simulink library "Yaw_Motor_Lib"  (Simulink 7.9)
settings: Solver=ode45  StartTime=0.0  StopTime=10.0  RelTol=1e-3
undefined symbols (not defined in the file): deg, gcbh, mech_rtmsupport, mech_support, s, WT_Params
libraries: fl_lib x7, mblibv1 x6, nesl_utility x5, elec_lib x1, Yaw_Gearbox_Lib x1
Description:
  | Copyright 2011 MathWorks, Inc.
settings Model: Creator=smiller  LastModifiedBy=smiller

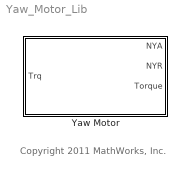
== system Yaw_Motor_Lib ==
  note: Copyright 2011 MathWorks, Inc.
  Yaw Motor : Subsystem
      mask Display: image(imread('Yaw_Servomotor_Horizontal_IMAGE.jpg'));

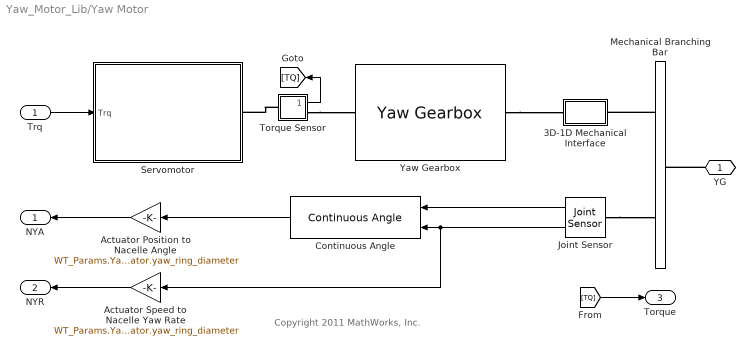
== system Yaw_Motor_Lib/Yaw Motor ==
  note: Copyright 2011 MathWorks, Inc.
  Trq : Inport
  3D-1D Mechanical Interface : Subsystem
  Actuator Position to Nacelle Angle : Gain  Gain=WT_Params.Yaw_Actuator.yaw_gear_diameter/WT_Params.Yaw_Actuator.yaw_ring_diameter
  Actuator Speed to Nacelle Yaw Rate : Gain  Gain=WT_Params.Yaw_Actuator.yaw_gear_diameter/WT_Params.Yaw_Actuator.yaw_ring_diameter
  Continuous Angle : mblibv1/Utilities/Continuous Angle  rad=deg  rads=deg/s
  Joint Sensor : mblibv1/Sensors &  Actuators/Joint Sensor  UpdateFromCAD=off  PhysicalDomain=Mechanical  PortType=blob  Muxed=off  Pose=off  Angle=on  AngleUnits=deg  ArcVelocity=on  ArcVelocityUnits=deg/s  ArcAcceleration=off  ArcAccelerationUnits=deg/s^2  CoordPosition=on  CoordPositionUnits=m  Velocity=off  VelocityUnits=m/s  Acceleration=off  AccelerationUnits=m/s^2  Quaternion=on  QuaternionDT=off  QuaternionDDT=off  QuaternionUnits=off  OutputVector=[1]  ActiveIO=off  Width=2  DialogClass=MechanicalSensorBlock  Primitive=R1  Force=off  ForceUnits=N  Torque=off  TorqueUnits=N*m  ReferenceFrame=Absolute (World)  ReactionSensedSide=Base  ReactionReferenceFrame=Local (Body CS)  ReactionForce=off  ReactionForceUnits=N  ReactionMoment=off  ReactionMomentUnits=N*m
  Mechanical Branching Bar : mblibv1/Utilities/Mechanical Branching Bar  LConnTagsString=_newl0  RConnTagsString=SA0|SA1  UpdateFromCAD=off  DialogClass=MechanicalBranchingBarBlock  NumSAPorts=2
  Servomotor : Subsystem
      mask Display: image(imread('Yaw_Servomotor_IMAGE.jpg'));
  Torque Sensor : Subsystem
      mask Display: disp('S')
  Yaw Gearbox : Yaw_Gearbox_Lib/Yaw Gearbox  SystemSampleTime=-1
  YG : PMIOPort  Port=1  Side=Right
  NYA : Outport
  NYR : Outport  Port=2
  Torque : Outport  Port=3
  wires:
  Trq/1 -> Servomotor/1(Trq)
  Joint Sensor/2 -> Actuator Speed to Nacelle Yaw Rate/1, Continuous Angle/2
  Joint Sensor/1 -> Continuous Angle/1
  Continuous Angle/1 -> Actuator Position to Nacelle Angle/1
  Actuator Position to Nacelle Angle/1 -> NYA/1
  Actuator Speed to Nacelle Yaw Rate/1 -> NYR/1
  Torque Sensor/1(Trq) -> [TQ]
  [TQ] -> Torque/1
  connections:
  Mechanical Branching Bar/RConn1 -- 3D-1D Mechanical Interface/RConn1
  Joint Sensor/LConn1 -- Mechanical Branching Bar/RConn2
  YG/RConn1 -- Mechanical Branching Bar/LConn1
  Torque Sensor/LConn1 -- Servomotor/RConn1
  Torque Sensor/RConn1 -- Yaw Gearbox/LConn1
  Yaw Gearbox/RConn1 -- 3D-1D Mechanical Interface/LConn1

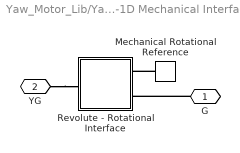
== system Yaw_Motor_Lib/Yaw Motor/3D-1D Mechanical Interface ==
  Mechanical Rotational Reference : fl_lib/Mechanical/Rotational Elements/Mechanical Rotational Reference  t_Log=off  LocalVarNames=|t  LocalVarDescs=|t  LocalVarLogging=0
  Revolute - Rotational Interface : Subsystem  DialogController=MECH.DynMechDlgSource  LoadFcn=mech_rtmsupport('LoadFcn',gcbh);mech_support('LoadFcn',gcbh);  StartFcn=mech_support('StartFcn',gcbh);  StopFcn=mech_support('StopFcn',gcbh);  mask(Revolute - Rotational Interface){UpdateFromCAD=off, PMImportedID=, ClassName=RevoluteRotationalInterface, DialogClass=RevoluteRotationalInterface, Primitive=R1}
      mask prompts: UpdateFromCAD "UPDATE_FROM_CAD"; PMImportedID "PMIMPORTED_ID"; Primitive "Connected to primitive :"
      mask help:
      | Connects a revolute primitive in the Joint attached at port R to any two mechanical rotational nodes in a Simscape network. Exchanges rotational kinetic energy between a machine and a network without loss. The base (B) and follower (F) ports correspond to the same ports on the Joint. Connect to Joint block to see Connected to primitive list.
      |
      | To ensure model validity, do not place inertia elements in interfaced Simscape circuit.
      mask init:
      | mech_preinitmask ();
      | mech_support('MaskInit',gcbh)
      settings: CopyFcn=mech_rtmsupport('CopyFcn',gcbh);mech_support('CopyFcn',gcbh);  DeleteFcn=mech_rtmsupport('DeleteFcn',gcbh);mech_support('DeleteFcn',gcbh);  UndoDeleteFcn=mech_support('UndoDeleteFcn',gcbh);  ModelCloseFcn=mech_rtmsupport('ModelCloseFcn',gcbh);mech_support('ModelCloseFcn',gcbh);  PreSaveFcn=mech_rtmsupport('PreSaveFcn',gcbh);  PostSaveFcn=mech_rtmsupport('PostSaveFcn',gcbh);  NameChangeFcn=mech_support('NameChangeFcn',gcbh);  PreCopyFcn=mech_rtmsupport('PreCopyFcn',gcbh);  CloseFcn=mech_support('CloseFcn',gcbh);  PreDeleteFcn=mech_rtmsupport('PreDeleteFcn',gcbh);
      mask Help: web(mech_help('revoluterotationalinterface'))
      mask Display: image(mech_getIcon('revolute_interface.bmp', 'Mechanical'),'center','on');color('magenta');port_label('lconn',1,'B');port_label('lconn',2,'F');color('black');port_label('rconn',1,'R');
  G : PMIOPort  Port=1  Side=Left
  YG : PMIOPort  Port=2  Side=Right
  connections:
  G/RConn1 -- Revolute - Rotational Interface/LConn2
  Mechanical Rotational Reference/LConn1 -- Revolute - Rotational Interface/LConn1
  YG/RConn1 -- Revolute - Rotational Interface/RConn1

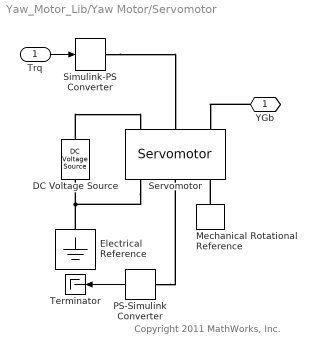
== system Yaw_Motor_Lib/Yaw Motor/Servomotor ==
  note: Copyright 2011 MathWorks, Inc.
  Trq : Inport
  DC Voltage Source : fl_lib/Electrical/Electrical Sources/DC Voltage Source  v0=WT_Params.Yaw_Actuator.Motor.voltage V  i_Log=off  v_Log=off  LocalVarNames=|current|voltage|power  LocalVarDescs=|Current (A)|Voltage (V)|Power (W)  LocalVarLogging=[0 0 0]
  Electrical Reference : fl_lib/Electrical/Electrical Elements/Electrical Reference  i_Log=off  LocalVarNames=|i  LocalVarDescs=|i  LocalVarLogging=[]
  Mechanical Rotational Reference : fl_lib/Mechanical/Rotational Elements/Mechanical Rotational Reference  t_Log=off  LocalVarNames=|t  LocalVarDescs=|t  LocalVarLogging=[]
  PS-Simulink Converter : nesl_utility/PS-Simulink Converter  PhysicalDomain=network_engine_domain  LeftPortType=input  RightPortType=output  SubClassName=ps_output  Unit=deg/s  AffineConversion=off
  Servomotor : elec_lib/Actuators & Drivers/Rotational Actuators/Servomotor  w_t=WT_Params.Yaw_Actuator.Motor.max_speed_vector  T_t=WT_Params.Yaw_Actuator.Motor.max_torque_vector  Tc=WT_Params.Yaw_Actuator.Motor.control_time_constant s  eff=100  w_eff=3.75e+03 rpm  T_eff=0.08 N*m  Pbase=0 W  Res=WT_Params.Yaw_Actuator.Motor.resistance Ohm  J=0 kg*m^2  lam=WT_Params.Yaw_Actuator.Motor.damping N*m/(rad/s)  speed0=0 rpm  LocalVarLogging=[]  alpha=0.00393 1/K  Tmeas=25 C  thermal_mass=100 J/K  initial_temperature=25 C
  Simulink-PS Converter : nesl_utility/Simulink-PS Converter  PhysicalDomain=network_engine_domain  LeftPortType=input  RightPortType=output  SubClassName=ps_input  Unit=1  AffineConversion=off  InputFilterTimeConstant=.001  UdotUserProvided=0  SimscapeFilterOrder=1  InputFiltering=off
  Terminator : Terminator
  YGb : PMIOPort  Port=1  Side=Right
  wires:
  PS-Simulink Converter/1 -> Terminator/1
  Trq/1 -> Simulink-PS Converter/1
  connections:
  DC Voltage Source/LConn1 -- Servomotor/LConn1
  Servomotor/RConn1 -- DC Voltage Source/RConn1 -- Electrical Reference/LConn1
  Mechanical Rotational Reference/LConn1 -- Servomotor/RConn3
  PS-Simulink Converter/LConn1 -- Servomotor/RConn2
  Simulink-PS Converter/RConn1 -- Servomotor/LConn2
  YGb/RConn1 -- Servomotor/LConn3

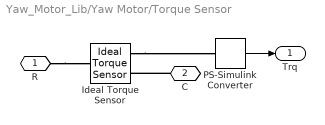
== system Yaw_Motor_Lib/Yaw Motor/Torque Sensor ==
  Ideal Torque Sensor : fl_lib/Mechanical/Mechanical Sensors/Ideal Torque Sensor  w_Log=off  t_Log=off  LocalVarNames=|w|t  LocalVarDescs=|w|t  LocalVarLogging=[0 0]
  PS-Simulink Converter : nesl_utility/PS-Simulink Converter  SystemSampleTime=-1  PhysicalDomain=network_engine_domain  LeftPortType=input  RightPortType=output  SubClassName=ps_output  Unit=1  AffineConversion=off
  R : PMIOPort  Port=1  Side=Left
  C : PMIOPort  Port=2  Side=Right
  Trq : Outport
  wires:
  PS-Simulink Converter/1 -> Trq/1
  connections:
  R/RConn1 -- Ideal Torque Sensor/LConn1
  C/RConn1 -- Ideal Torque Sensor/RConn1
  Ideal Torque Sensor/RConn2 -- PS-Simulink Converter/LConn1

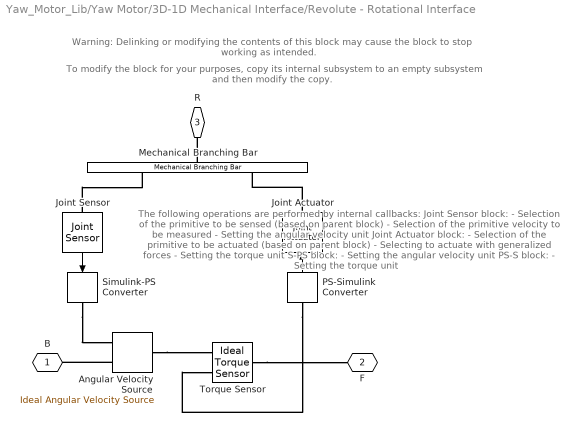
== system Yaw_Motor_Lib/Yaw Motor/3D-1D Mechanical Interface/Revolute - Rotational Interface ==
  note: Warning: Delinking or modifying the contents of
      | this block may cause the block to stop working as intended.
  note: To modify the block for your purposes, copy its internal subsystem
      | to an empty subsystem and then modify the copy.
  note: The following operations are performed by internal callbacks:
      |
      | Joint Sensor block:
      |    - Selection of the primitive to be sensed (based on parent block)
      |    - Selection of the primitive velocity to be measured
      |    - Setting the angular velocity unit
      |
      | Joint Actuator block:
      |    - Selection of the primitive to be actuated (based on parent block)
      |    - Selecting to actuate with generalized forces
      |    - Setting the torque unit
      |
      | S-PS block:
      |    - Setting the angular velocity unit
      |
      | PS-S block:
      |    - Setting the torque unit
  Angular Velocity Source : fl_lib/Mechanical/Mechanical Sources/Ideal Angular Velocity Source  w_Log=off  t_Log=off  LocalVarNames=|torque|rel_velocity|power  LocalVarDescs=|Torque (N*m)|Relative velocity (rad/s)|Power generated by the sourcec(W)  LocalVarLogging=[0 0 0]
  Joint Actuator : mblibv1/Sensors &  Actuators/Joint Actuator  UpdateFromCAD=off  PhysicalDomain=Mechanical  PortType=blob  ActuationStyle=Force  AngleUnits=deg  ArcVelocityUnits=deg/s  ArcAccelerationUnits=deg/s^2  CoordPositionUnits=m  VelocityUnits=m/s  AccelerationUnits=m/s^2  ForceUnits=N  TorqueUnits=N*m  ActiveIO=off  Width=1  DialogClass=MechanicalActuatorBlock  Primitive=R1  ReferenceFrame=Absolute (World)
  Joint Sensor : mblibv1/Sensors &  Actuators/Joint Sensor  UpdateFromCAD=off  PhysicalDomain=Mechanical  PortType=blob  Muxed=on  Pose=off  Angle=off  AngleUnits=deg  ArcVelocity=on  ArcVelocityUnits=rad/s  ArcAcceleration=off  ArcAccelerationUnits=deg/s^2  CoordPosition=off  CoordPositionUnits=m  Velocity=off  VelocityUnits=m/s  Acceleration=off  AccelerationUnits=m/s^2  Quaternion=off  QuaternionDT=off  QuaternionDDT=off  QuaternionUnits=off  OutputVector=[1]  ActiveIO=off  Width=1  DialogClass=MechanicalSensorBlock  Primitive=R1  Force=off  ForceUnits=N  Torque=off  TorqueUnits=N*m  ReferenceFrame=Absolute (World)  ReactionSensedSide=Base  ReactionReferenceFrame=Absolute (World)  ReactionForce=off  ReactionForceUnits=N  ReactionMoment=off  ReactionMomentUnits=N*m
  Mechanical Branching Bar : mblibv1/Utilities/Mechanical Branching Bar  LConnTagsString=_newl0  RConnTagsString=SA0|SA1  UpdateFromCAD=off  DialogClass=MechanicalBranchingBarBlock  NumSAPorts=2
  PS-Simulink Converter : nesl_utility/PS-Simulink Converter  PhysicalDomain=network_engine_domain  LeftPortType=input  RightPortType=output  SubClassName=ps_output  Unit=N*m  AffineConversion=off
  Simulink-PS Converter : nesl_utility/Simulink-PS Converter  PhysicalDomain=network_engine_domain  LeftPortType=input  RightPortType=output  SubClassName=ps_input  Unit=rad/s  AffineConversion=off  InputFilterTimeConstant=.001  UdotUserProvided=1  SimscapeFilterOrder=1  InputFiltering=on
  Torque Sensor : fl_lib/Mechanical/Mechanical Sensors/Ideal Torque Sensor  w_Log=off  t_Log=off  LocalVarNames=|w|t  LocalVarDescs=|w|t  LocalVarLogging=[]
  B : PMIOPort  Port=1  Side=Left
  F : PMIOPort  Port=2  Side=Left
  R : PMIOPort  Port=3  Side=Right
  wires:
  PS-Simulink Converter/1 -> Joint Actuator/1
  Joint Sensor/1 -> Simulink-PS Converter/1
  connections:
  Joint Actuator/RConn1 -- Mechanical Branching Bar/RConn2
  Joint Sensor/LConn1 -- Mechanical Branching Bar/RConn1
  Mechanical Branching Bar/LConn1 -- R/RConn1
  Torque Sensor/LConn1 -- F/RConn1
  Simulink-PS Converter/RConn1 -- Angular Velocity Source/RConn1
  Angular Velocity Source/RConn2 -- B/RConn1
  Angular Velocity Source/LConn1 -- Torque Sensor/RConn1
  PS-Simulink Converter/LConn1 -- Torque Sensor/RConn2
